simulink library "mbrt_lib_level0"  (R2026a)
settings: Solver=VariableStepAuto
settings Model: Creator=ftraenkle  LastModifiedBy=thele

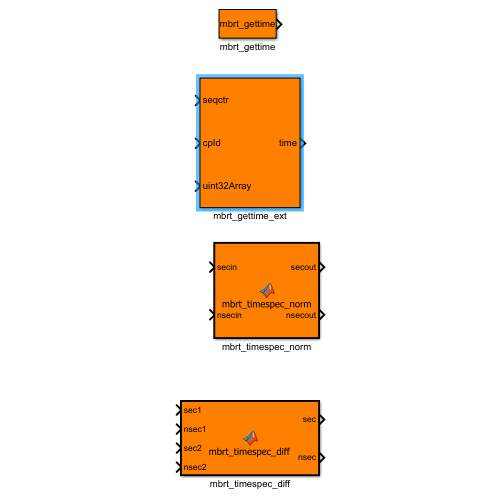
[thumbnail: Simulink's stored preview of the top-level diagram]
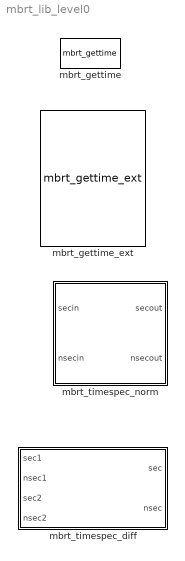
== system mbrt_lib_level0 ==
  mbrt_gettime : S-Function  FunctionName=mbrt_gettime  SFunctionDeploymentMode=off  EnableBusSupport=off
  mbrt_gettime_ext : S-Function  FunctionName=mbrt_gettime_ext  SFunctionDeploymentMode=off  EnableBusSupport=off
      mask Display:
      | port_label('input', 1, 'seqctr');
      | port_label('input', 2, 'cpId');
      | port_label('input', 3, 'uint32Array');
      | port_label('output', 1, 'time');
  mbrt_timespec_diff : MATLAB Function  TreatAsAtomicUnit=on
  mbrt_timespec_norm : MATLAB Function  TreatAsAtomicUnit=on

== matlab function mbrt_lib_level0/mbrt_timespec_norm ==
  data: secin input; secout output; nsecin input; nsecout output
function [ secout, nsecout ] = mbrt_timespec_norm(secin, nsecin)

if ~isa(secin, 'int32')
    error('secin must be int32');
end
if ~isa(nsecin, 'int32')
    error('nsecin must be int32');
end
%% normalize
nsec_sec = idivide(nsecin, int32(1000000000), 'floor');
secout = secin + nsec_sec;
%nsec = int32(int64(nsecin) - int64(1000000000) * int64(nsec_sec));
nsecout = nsecin - 1000000000 * nsec_sec;
end

== matlab function mbrt_lib_level0/mbrt_timespec_diff ==
  data: sec1 input; sec output; nsec1 input; sec2 input; nsec2 input; nsec output
function [ sec, nsec ] = mbrt_timespec_diff(sec1, nsec1, sec2, nsec2)

%% normalize
[ sec1norm, nsec1norm ] = timespec_norm(sec1, nsec1);
[ sec2norm, nsec2norm ] = timespec_norm(sec2, nsec2);
[ sec, nsec ] = timespec_norm(sec1norm - sec2norm, nsec1norm - nsec2norm);
end

%% auxiliary function
function [ secout, nsecout ] = timespec_norm(secin, nsecin)

if ~isa(secin, 'int32')
    error('secin must be int32');
end
if ~isa(nsecin, 'int32')
    error('nsecin must be int32');
end
%% normalize
nsec_sec = idivide(nsecin, int32(1000000000), 'floor');
secout = secin + nsec_sec;
%nsec = int32(int64(nsecin) - int64(1000000000) * int64(nsec_sec));
nsecout = nsecin - 1000000000 * nsec_sec;
end
